simulink model "svm_stc_bldc"  (R2021a)
settings: Solver=VariableStepAuto  StartTime=0.0  StopTime=t_sim  FixedStep=t_int  MinStep=1e-6  RelTol=1e-3  EnableMultiTasking=on
InitFcn:
  | svm_stc_bldc_data
values from neighbouring files (symbols this model uses):
  b = T_nom/Q_nom    (= 6.18430636014)    [bldc_data.m]
  flux_obs_gain = 4e4    (= 40000)    [bldc_data.m]
  Id = Iq    [i_loop_data.m]
  Jm = 0.3*0.05^2    (= 0.00075)    [bldc_data.m]
  theta_obs_gain = 2e6    (= 2000000)    [bldc_data.m]
  Vcc = 360    [bldc_data.m]
undefined symbols (not defined in the file or in its folder): fluid, i_sns, Iq, p, pmsm, r, speed_obs, v_stc
libraries: mcbcontrolslib x4, simulink x2, pid_lib x1, autolibpmsmexterior x1
settings Model: Creator=Augusto  LastModifiedBy=Rodrigo
settings SolverCC: AlgebraicLoopSolver=TrustRegion  AutoInsertRateTranBlk=on
settings DataIOCC: LimitDataPoints=on  SaveFormat=Array  ReturnWorkspaceOutputs=off
settings OptimizationCC: LifeSpan=inf
settings DebuggingCC: UnderspecifiedInitializationDetection=Classic  MergeDetectMultiDrivingBlocksExec=none  SolverPrmCheckMsg=warning  SFUnexpectedBacktrackingDiag=warning  SFNoUnconditionalDefaultTransitionDiag=warning  SFExecutionAtInitializationDiag=none  ArithmeticOperatorsInVariantConditions=warning
settings HardwareCC: ProdBitPerPointer=32  ProdBitPerSizeT=32  ProdBitPerPtrDiffT=32  ProdLargestAtomicFloat=None  ProdIntDivRoundTo=Undefined  ProdEndianess=Unspecified  ProdWordSize=32  ProdHWDeviceType=32-bit Generic
settings ModelReferenceCC: PropagateSignalLabelsOutOfModel=off
settings SFSimCC: SimUseLocalCustomCode=off  CustomCodeUndefinedFunction=UseInterfaceOnly
settings RTWCC: RTWUseLocalCustomCode=off  DLArmComputeVersion=20.02.1
settings CodeAppCC: StateflowObjectComments=on
settings GRTTargetCC: TargetLangStandard=C89/C90 (ANSI)
settings ConfigComp: CovMetricSettings=dw  CovSaveCumulativeToWorkspaceVar=on  CovSaveSingleToWorkspaceVar=on  CovExternalEMLEnable=off

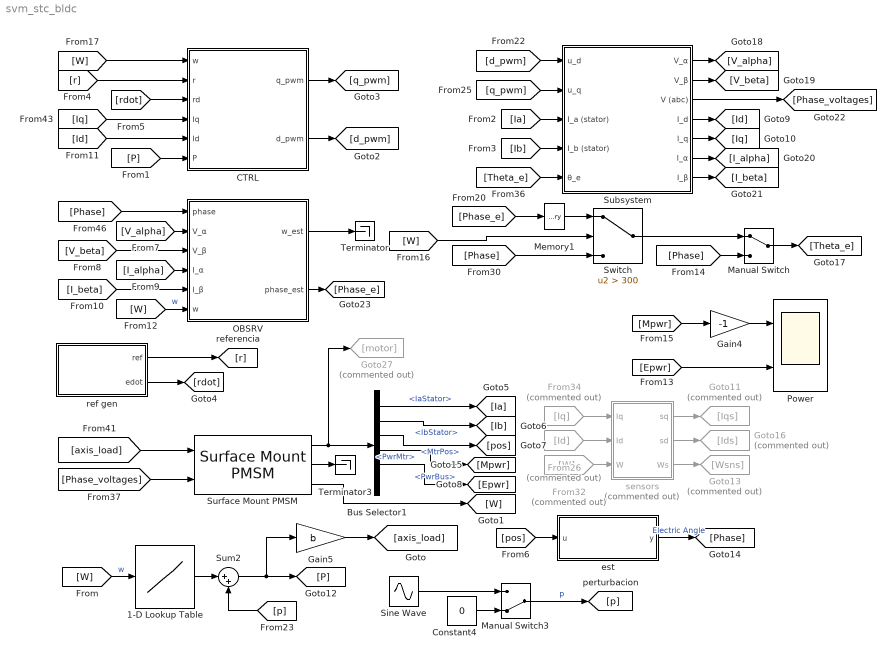
== system svm_stc_bldc ==
  1-D Lookup Table : Lookup_n-D  NumberOfTableDimensions=1  BreakpointsForDimension1=fluid.W  Table=fluid.P  InternalRulePriority=Speed  RndMeth=Simplest  InputSameDT=on
  Bus Selector1 : BusSelector  OutputSignals=IaStator,IbStator,MtrPos,PwrInfo.PwrTrnsfrd.PwrMtr,PwrInfo.PwrTrnsfrd.PwrBus,MtrSpd
  CTRL : Subsystem
  Constant4 : Constant  Value=0
  From26 : From  Commented=on  GotoTag=Id
  From32 : From  Commented=on  GotoTag=W
  From34 : From  Commented=on  GotoTag=Iq
  Gain4 : Gain  Gain=-1
  Gain5 : Gain  Gain=b
  Goto11 : Goto  Commented=on  GotoTag=Iqs
  Goto13 : Goto  Commented=on  GotoTag=Wsns
  Goto16 : Goto  Commented=on  GotoTag=Ids
  Goto27 : Goto  Commented=on  GotoTag=motor
  Manual Switch : ManualSwitch
  Manual Switch3 : ManualSwitch  CurrentSetting=0
  Memory1 : Memory
  OBSRV : Subsystem
  Power : Scope  NumInputPorts=2
  Sine Wave : Sin  Amplitude=p.a  Frequency=p.w  SampleTime=0
  Subsystem : Subsystem
  Sum2 : Sum  Inputs=|++
  Surface Mount PMSM : autolibpmsmexterior/Surface Mount PMSM  port_config=Torque  sim_type=Continuous  Ts=0.001  P=pmsm.spec.poles/2  Rs=pmsm.perf.Rs  Ldq_=pmsm.perf.L  KConstText=Permanent flux linkage constant (lambda_pm):  lambda_pm=pmsm.perf.phi  Ke=159.9771  Kt=1.323  mechanical=[Jm, 0.0001, 0.2]  idq0=[0 0]  theta_init=0  omega_init=Wo  KConst=pmsm.perf.phi  lambda_pm_calc=pmsm.perf.phi  RefBlkName='autolibpmsmexterior/Surface Mount PMSM'  aMode=5  Ldq="[0.0017      0.0017]"
      settings: SourceProductBaseCode=PW,DR,MT,UV,VE
  Switch : Switch  Criteria=u2 > Threshold  Threshold=300
  Terminator : Terminator
  Terminator3 : Terminator
  est : MATLAB Function  TreatAsAtomicUnit=on
  ref gen : Subsystem
  sensors : Subsystem  Commented=on
  wires:
  1-D Lookup Table/1 -> Sum2/1
  [p] -> Sum2/2
  Sum2/1 -> Gain5/1, [P]
  Sine Wave/1 -> Manual Switch3/1
  Manual Switch3/1 -> [p]  "p"
  Constant4/1 -> Manual Switch3/2
  [W] -> 1-D Lookup Table/1  "w"
  From34/1 -> sensors/1(Iq)
  sensors/1(sq) -> Goto11/1
  From32/1 -> sensors/3(W)
  [Phase_voltages] -> Surface Mount PMSM/2
  Bus Selector1/2 -> [Ib]  "<IbStator>"
  Subsystem/1(V_α) -> [V_alpha]
  [axis_load] -> Surface Mount PMSM/1
  [Theta_e] -> Subsystem/5(θ_e)
  Subsystem/2(V_β) -> [V_beta]
  Bus Selector1/1 -> [Ia]  "<IaStator>"
  Subsystem/6(I_α) -> [I_alpha]
  Subsystem/5(I_q) -> [Iq]
  Subsystem/7(I_β) -> [I_beta]
  Subsystem/4(I_d) -> [Id]
  est/1(y) -> [Phase]  "Electric Angle"
  Bus Selector1/3 -> [pos]  "<MtrPos>"
  Subsystem/3(V (abc)) -> [Phase_voltages]
  Surface Mount PMSM/1 -> Goto27/1, Bus Selector1/1
  Surface Mount PMSM/2 -> Terminator3/1
  Gain5/1 -> [axis_load]
  From26/1 -> sensors/2(Id)
  [Phase] -> OBSRV/1(phase)
  [d_pwm] -> Subsystem/1(u_d)
  [q_pwm] -> Subsystem/2(u_q)
  [W] -> CTRL/1(w)
  [r] -> CTRL/2(r)
  [rdot] -> CTRL/3(rd)
  [Iq] -> CTRL/4(Iq)
  [Id] -> CTRL/5(Id)
  CTRL/1(q_pwm) -> [q_pwm]
  CTRL/2(d_pwm) -> [d_pwm]
  [P] -> CTRL/6(P)
  [Ia] -> Subsystem/3(I_a (stator))
  [Ib] -> Subsystem/4(I_b (stator))
  [pos] -> est/1(u)
  sensors/2(sd) -> Goto16/1
  sensors/3(Ws) -> Goto13/1
  ref gen/1(ref) -> [r]
  ref gen/2(edot) -> [rdot]
  [V_alpha] -> OBSRV/2(V_α)
  [V_beta] -> OBSRV/3(V_β)
  [I_alpha] -> OBSRV/4(I_α)
  [I_beta] -> OBSRV/5(I_β)
  [W] -> OBSRV/6(w)  "w"
  [Epwr] -> Power/2
  [Mpwr] -> Gain4/1
  Gain4/1 -> Power/1
  Bus Selector1/5 -> [Epwr]  "<PwrBus>"
  Bus Selector1/4 -> [Mpwr]  "<PwrMtr>"
  OBSRV/2(phase_est) -> [Phase_e]
  OBSRV/1(w_est) -> Terminator/1
  [W] -> Switch/2
  Switch/1 -> Manual Switch/1
  [Phase] -> Switch/3
  Manual Switch/1 -> [Theta_e]
  [Phase] -> Manual Switch/2
  Surface Mount PMSM/3 -> [W]
  [Phase_e] -> Memory1/1
  Memory1/1 -> Switch/1

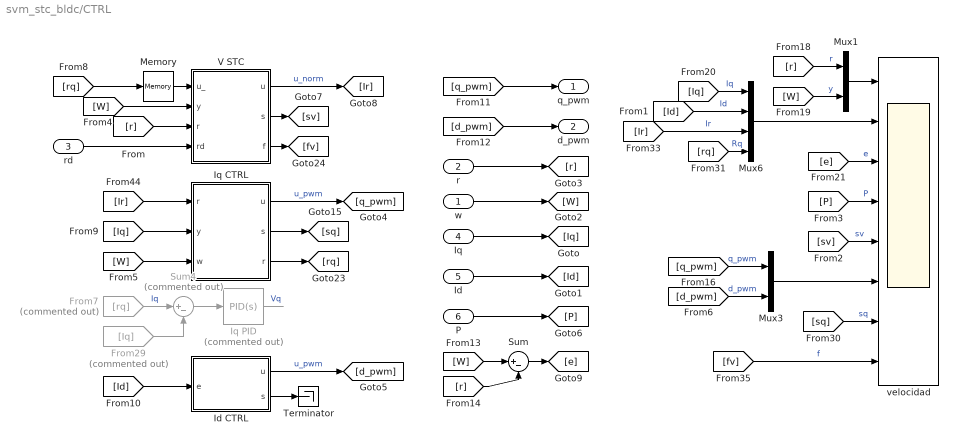
== system svm_stc_bldc/CTRL ==
  w : Inport
  r : Inport  Port=2
  rd : Inport  Port=3
  Iq : Inport  Port=4
  Id : Inport  Port=5
  P : Inport  Port=6
  From29 : From  Commented=on  GotoTag=Iq
  From7 : From  Commented=on  GotoTag=rq
  Id CTRL : MATLAB Function  TreatAsAtomicUnit=on  SystemSampleTime=Id.ts
  Iq CTRL : MATLAB Function  TreatAsAtomicUnit=on  SystemSampleTime=Iq.ts
  Iq PID : pid_lib/PID Controller  Commented=on  Controller=PID  Form=Parallel  TimeDomain=Continuous-time  UseExternalTs=off  SampleTime=-1  IntegratorMethod=Forward Euler  FilterMethod=Forward Euler  ControllerParametersSource=internal  P=10/Vcc  I=100/Vcc  D=1/Vcc  UseFilter=on  N=100  TunerSelectOption=Transfer Function Based (PID Tuner App)  InitialConditionSource=internal  InitialConditionForIntegrator=0  InitialConditionForFilter=0  DifferentiatorICPrevScaledInput=0  ExternalReset=none  TrackingMode=off  Kt=1  LimitOutput=on  SatLimitsSource=internal  UpperSaturationLimit=Vcc  LowerSaturationLimit=-Vcc  LinearizeAsGain=on  AntiWindupMode=back-calculation  Kb=1  POutMin=[]  POutMax=[]  IOutMin=[]  IOutMax=[]  DOutMin=[]  DOutMax=[]  NOutMin=[]  NOutMax=[]  SumOutMin=[]  SumOutMax=[]  SaturationOutMin=[]  SaturationOutMax=[]  PParamMin=[]  PParamMax=[]  IParamMin=[]  IParamMax=[]  DParamMin=[]  DParamMax=[]  NParamMin=[]  NParamMax=[]  KbParamMin=[]  KbParamMax=[]  KtParamMin=[]  KtParamMax=[]  KbOutMin=[]  KbOutMax=[]  KtOutMin=[]  KtOutMax=[]  IntegratorOutMin=[]  IntegratorOutMax=[]  FilterOutMin=[]  FilterOutMax=[]  SumI1OutMin=[]  SumI1OutMax=[]  SumI2OutMin=[]  SumI2OutMax=[]  SumI3OutMin=[]  SumI3OutMax=[]  SumI4OutMin=[]  SumI4OutMax=[]  SumDOutMin=[]  SumDOutMax=[]  DifferentiatorOutMin=[]  DifferentiatorOutMax=[]  FilterDiffOutCoefMin=[]  FilterDiffOutCoefMax=[]  ReciprocalOutMin=[]  ReciprocalOutMax=[]  SumDenOutMin=[]  SumDenOutMax=[]  SumNumOutMin=[]  SumNumOutMax=[]  DivideOutMin=[]  DivideOutMax=[]  UdiffTsProdOutMin=[]  UdiffTsProdOutMax=[]  NTsProdOutMin=[]  NTsProdOutMax=[]  UintegralTsProdOutMin=[]  UintegralTsProdOutMax=[]  UngainTsProdOutMin=[]  UngainTsProdOutMax=[]  IntegratorContinuousStateAttributes=''  IntegratorStateMustResolveToSignalObject=off  IntegratorRTWStateStorageClass=Auto  FilterContinuousStateAttributes=''  FilterStateMustResolveToSignalObject=off  FilterRTWStateStorageClass=Auto  ParallelPVariant=InternalParameters  IdealPVariant=Disabled  IVariant=InternalParameters  DVariant=InternalParameters  IntegratorVariant=Continuous  SatVariant=Enabled  AWVariant=BackCalculation  PCopyVariant=Disabled  TRVariant=Disabled  FdbkBlocksVariant=Forward  IdealPFdbkVariant=Disabled  SatFdbkVariant=Disabled  DerivativeFilterVariant=ContFilter  NVariant=InternalParameters  NCopyVariant=Disabled  FilterICVariant=InternalICsFilter  IntegratorICVariant=InternalICs  ExternalResetVariant=Disabled  TRSumVariant=Passthrough  SumFdbkVariant=Disabled  SumVariant=Sum_PID  TsampFilterVariant=InternalTs  TsampNgainVariant=Passthrough  TsampIntegralVariant=Passthrough  ExternalSaturationOutDataTypeStr=Inherit: Same as second input
  Memory : Memory
  Mux1 : Mux  Inputs=2
  Mux3 : Mux  Inputs=2
  Mux6 : Mux
  Sum : Sum  Inputs=|+-
  Sum4 : Sum  Commented=on  Inputs=|+-
  Terminator : Terminator
  V STC : MATLAB Function  TreatAsAtomicUnit=on  SystemSampleTime=v_stc.ts
  velocidad : Scope  NumInputPorts=8
  q_pwm : Outport
  d_pwm : Outport  Port=2
  wires:
  V STC/3(f) -> [fv]
  Sum4/1 -> Iq PID/1
  From29/1 -> Sum4/2
  Id/1 -> [Id]
  V STC/2(s) -> [sv]
  Memory/1 -> V STC/1(u_)
  Id CTRL/1(u) -> [d_pwm]  "u_pwm"
  [Ir] -> Iq CTRL/1("r ")
  r/1 -> [r]
  Iq CTRL/1(u) -> [q_pwm]  "u_pwm"
  [rq] -> Memory/1
  Iq PID/1 -> ?  "Vq"
  Iq CTRL/3(r) -> [rq]
  w/1 -> [W]
  From7/1 -> Sum4/1  "Iq"
  V STC/1(u) -> [Ir]  "u_norm"
  Id CTRL/2(s) -> Terminator/1
  Iq/1 -> [Iq]
  rd/1 -> V STC/4(rd)
  Iq CTRL/2(s) -> [sq]
  [sq] -> velocidad/7  "sq"
  [sv] -> velocidad/5  "sv"
  [W] -> Mux1/2  "y"
  [rq] -> Mux6/4  "Rq"
  [P] -> velocidad/4  "P"
  [d_pwm] -> Mux3/2  "d_pwm"
  [e] -> velocidad/3  "e"
  [Ir] -> Mux6/3  "Ir"
  [Id] -> Mux6/2  "Id"
  Mux6/1 -> velocidad/2
  [fv] -> velocidad/8  "f"
  Mux1/1 -> velocidad/1
  [q_pwm] -> Mux3/1  "q_pwm"
  [r] -> Mux1/1  "r"
  Mux3/1 -> velocidad/6
  [Iq] -> Mux6/1  "Iq"
  [r] -> V STC/3(r)
  [W] -> V STC/2(y)
  [W] -> Iq CTRL/3(w)
  [Iq] -> Iq CTRL/2(y)
  [Id] -> Id CTRL/1(e)
  [q_pwm] -> q_pwm/1
  [d_pwm] -> d_pwm/1
  P/1 -> [P]
  Sum/1 -> [e]
  [W] -> Sum/1
  [r] -> Sum/2

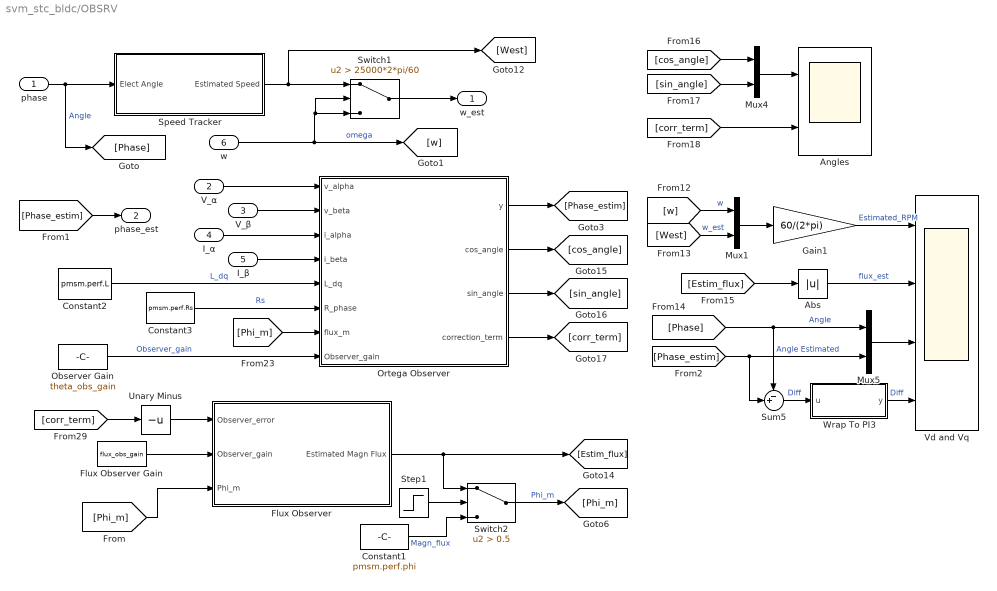
== system svm_stc_bldc/OBSRV ==
  phase : Inport
  V_α : Inport  Port=2
  V_β : Inport  Port=3
  I_α : Inport  Port=4
  I_β : Inport  Port=5
  w : Inport  Port=6
  Abs : Abs
  Angles : Scope  NumInputPorts=2
  Constant1 : Constant  Value=pmsm.perf.phi
  Constant2 : Constant  Value=pmsm.perf.L
  Constant3 : Constant  Value=pmsm.perf.Rs
  Flux Observer : Subsystem
  Flux Observer Gain : Constant  Value=flux_obs_gain
  Gain1 : Gain  Gain=60/(2*pi)
  Mux1 : Mux  Inputs=2
  Mux4 : Mux  Inputs=2
  Mux5 : Mux  Inputs=2
  Observer Gain : Constant  Value=theta_obs_gain
  Ortega Observer : Subsystem
  Speed Tracker : Subsystem
  Step1 : Step  Time=0.01  After=2  SampleTime=0
  Sum5 : Sum  Inputs=-+|
  Switch1 : Switch  Criteria=u2 > Threshold  Threshold=25000*2*pi/60
  Switch2 : Switch  Criteria=u2 > Threshold  Threshold=0.5
  Unary Minus : UnaryMinus
  Vd and Vq : Scope  NumInputPorts=4
  Wrap To PI3 : MATLAB Function  TreatAsAtomicUnit=on
  w_est : Outport
  phase_est : Outport  Port=2
  wires:
  Switch1/1 -> w_est/1
  [Phi_m] -> Ortega Observer/7(flux_m)
  V_β/1 -> Ortega Observer/2(v_beta)
  Ortega Observer/3(sin_angle) -> [sin_angle]
  Constant2/1 -> Ortega Observer/5(L_dq)  "L_dq"
  Constant3/1 -> Ortega Observer/6(R_phase)  "Rs"
  Ortega Observer/1(y) -> [Phase_estim]
  Ortega Observer/2(cos_angle) -> [cos_angle]
  Flux Observer/1(Estimated Magn Flux) -> Switch2/1, [Estim_flux]
  Constant1/1 -> Switch2/3  "Magn_flux"
  Unary Minus/1 -> Flux Observer/1(Observer_error)
  Step1/1 -> Switch2/2
  Flux Observer Gain/1 -> Flux Observer/2(Observer_gain)
  Observer Gain/1 -> Ortega Observer/8(Observer_gain)  "Observer_gain"
  V_α/1 -> Ortega Observer/1(v_alpha)
  Ortega Observer/4(correction_term) -> [corr_term]
  Switch2/1 -> [Phi_m]  "Phi_m"
  [corr_term] -> Unary Minus/1
  I_α/1 -> Ortega Observer/3(i_alpha)
  I_β/1 -> Ortega Observer/4(i_beta)
  phase/1 -> [Phase], Speed Tracker/1(Elect Angle)  "Angle"
  [Phi_m] -> Flux Observer/3(Phi_m)
  Mux4/1 -> Angles/1
  [w] -> Mux1/1  "w"
  [sin_angle] -> Mux4/2
  [cos_angle] -> Mux4/1
  [West] -> Mux1/2  "w_est"
  Abs/1 -> Vd and Vq/2  "flux_est"
  [Estim_flux] -> Abs/1
  [corr_term] -> Angles/2
  Mux1/1 -> Gain1/1
  [Phase_estim] -> phase_est/1
  Speed Tracker/1(Estimated Speed) -> [West], Switch1/1
  Gain1/1 -> Vd and Vq/1  "Estimated_RPM"
  [Phase] -> Sum5/1, Mux5/1  "Angle"
  Mux5/1 -> Vd and Vq/3
  [Phase_estim] -> Sum5/2, Mux5/2  "Angle Estimated"
  Sum5/1 -> Wrap To PI3/1(u)  "Diff"
  Wrap To PI3/1(y) -> Vd and Vq/4  "Diff"
  w/1 -> [w], Switch1/3, Switch1/2  "omega"

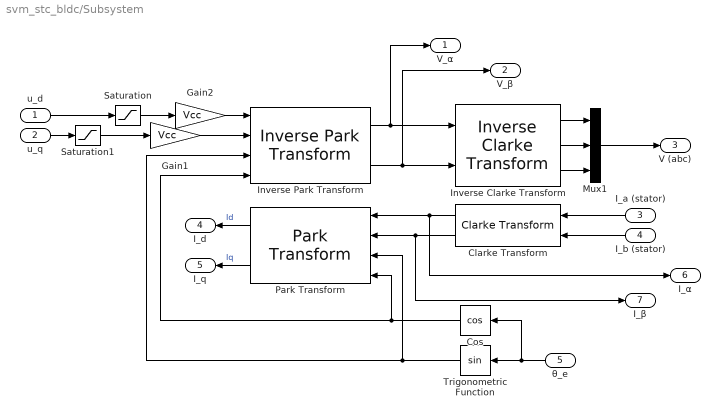
== system svm_stc_bldc/Subsystem ==
  u_d : Inport
  u_q : Inport  Port=2
  I_a (stator) : Inport  Port=3
  I_b (stator) : Inport  Port=4
  θ_e : Inport  Port=5
  Clarke Transform : mcbcontrolslib/Clarke Transform  VariantControl=Variant2
  Cos : Trigonometry  Operator=cos
  Gain1 : Gain  Gain=Vcc
  Gain2 : Gain  Gain=Vcc
  Inverse Clarke Transform : mcbcontrolslib/Inverse Clarke Transform
      settings: SourceProductBaseCode=MT
  Inverse Park Transform : mcbcontrolslib/Inverse Park Transform  AxisAlignment=D-axis
  Mux1 : Mux  Inputs=3
  Park Transform : mcbcontrolslib/Park Transform  AxisAlignment=D-axis
      settings: SourceProductBaseCode=MT
  Saturation : Saturate  UpperLimit=0.95  LowerLimit=-0.95
  Saturation1 : Saturate  UpperLimit=0.95  LowerLimit=-0.95
  Trigonometric Function : Trigonometry
  V_α : Outport
  V_β : Outport  Port=2
  V (abc) : Outport  Port=3
  I_d : Outport  Port=4
  I_q : Outport  Port=5
  I_α : Outport  Port=6
  I_β : Outport  Port=7
  wires:
  I_b (stator)/1 -> Clarke Transform/2
  Mux1/1 -> V (abc)/1
  u_q/1 -> Saturation1/1
  I_a (stator)/1 -> Clarke Transform/1
  Clarke Transform/2 -> I_β/1, Park Transform/2
  Cos/1 -> Park Transform/4, Inverse Park Transform/4
  Clarke Transform/1 -> I_α/1, Park Transform/1
  θ_e/1 -> Cos/1, Trigonometric Function/1
  Park Transform/2 -> I_q/1  "Iq"
  Inverse Park Transform/2 -> V_β/1, Inverse Clarke Transform/2
  Park Transform/1 -> I_d/1  "Id"
  Inverse Clarke Transform/2 -> Mux1/2
  Trigonometric Function/1 -> Park Transform/3, Inverse Park Transform/3
  u_d/1 -> Saturation/1
  Inverse Park Transform/1 -> V_α/1, Inverse Clarke Transform/1
  Inverse Clarke Transform/3 -> Mux1/3
  Inverse Clarke Transform/1 -> Mux1/1
  Gain2/1 -> Inverse Park Transform/1
  Gain1/1 -> Inverse Park Transform/2
  Saturation/1 -> Gain2/1
  Saturation1/1 -> Gain1/1

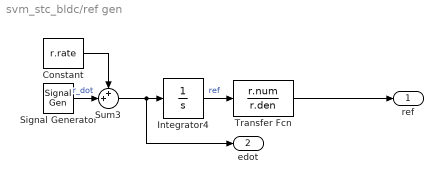
== system svm_stc_bldc/ref gen ==
  Constant : Constant  Value=r.rate
  Integrator4 : Integrator  InitialCondition=r.off  LimitOutput=on  UpperSaturationLimit=r.lim  LowerSaturationLimit=0
  Signal Generator : SignalGenerator  Amplitude=r.a  Frequency=r.f
  Sum3 : Sum  Inputs=++|
  Transfer Fcn : TransferFcn  Numerator=r.num  Denominator=r.den
  ref : Outport
  edot : Outport  Port=2
  wires:
  Constant/1 -> Sum3/1
  Signal Generator/1 -> Sum3/2  "r_dot"
  Sum3/1 -> edot/1, Integrator4/1
  Transfer Fcn/1 -> ref/1
  Integrator4/1 -> Transfer Fcn/1  "ref"

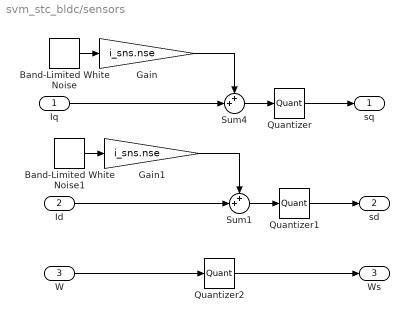
== system svm_stc_bldc/sensors ==
  Iq : Inport
  Id : Inport  Port=2
  W : Inport  Port=3
  Band-Limited White Noise : simulink/Sources/Band-Limited White Noise  Cov=Iq.ts  Ts=Iq.ts  seed=[29841]
  Band-Limited White Noise1 : simulink/Sources/Band-Limited White Noise  Cov=Iq.ts  Ts=Iq.ts  seed=[29841]
  Gain : Gain  Gain=i_sns.nse
  Gain1 : Gain  Gain=i_sns.nse
  Quantizer : Quantizer  QuantizationInterval=i_sns.qnt
  Quantizer1 : Quantizer  QuantizationInterval=i_sns.qnt
  Quantizer2 : Quantizer  QuantizationInterval=w_sns.qnt
  Sum1 : Sum  Inputs=++|
  Sum4 : Sum  Inputs=++|
  sq : Outport
  sd : Outport  Port=2
  Ws : Outport  Port=3
  wires:
  Iq/1 -> Sum4/2
  Band-Limited White Noise/1 -> Gain/1
  Sum4/1 -> Quantizer/1
  Quantizer/1 -> sq/1
  Gain/1 -> Sum4/1
  Band-Limited White Noise1/1 -> Gain1/1
  Quantizer1/1 -> sd/1
  Id/1 -> Sum1/2
  Sum1/1 -> Quantizer1/1
  Gain1/1 -> Sum1/1
  W/1 -> Quantizer2/1
  Quantizer2/1 -> Ws/1

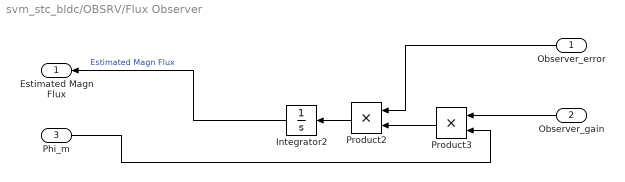
== system svm_stc_bldc/OBSRV/Flux Observer ==
  Observer_error : Inport
  Observer_gain : Inport  Port=2
  Phi_m : Inport  Port=3
  Integrator2 : Integrator
  Product2 : Product
  Product3 : Product
  Estimated Magn Flux : Outport
  wires:
  Product3/1 -> Product2/2
  Product2/1 -> Integrator2/1
  Observer_error/1 -> Product2/1
  Observer_gain/1 -> Product3/1
  Phi_m/1 -> Product3/2
  Integrator2/1 -> Estimated Magn Flux/1  "Estimated Magn Flux"

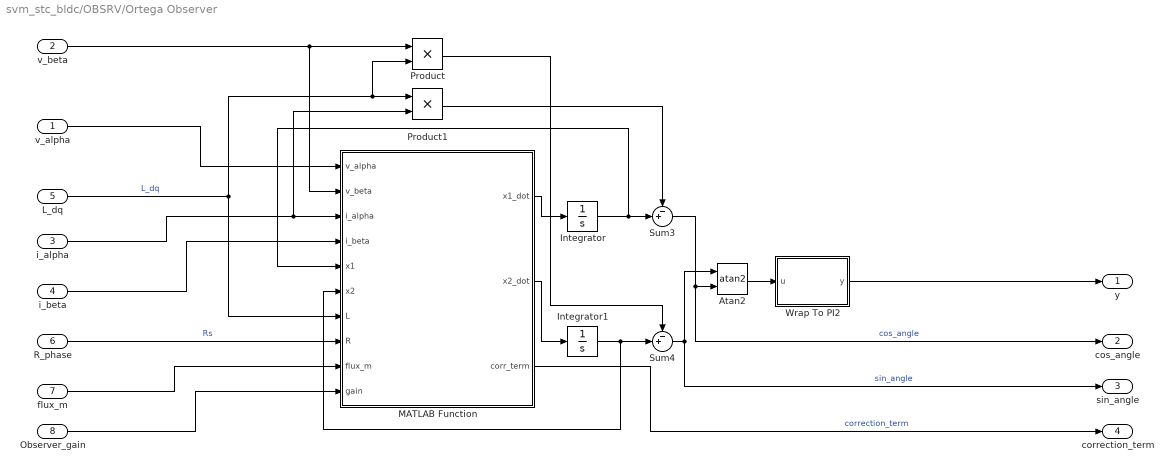
== system svm_stc_bldc/OBSRV/Ortega Observer ==
  v_alpha : Inport
  v_beta : Inport  Port=2
  i_alpha : Inport  Port=3
  i_beta : Inport  Port=4
  L_dq : Inport  Port=5
  R_phase : Inport  Port=6
  flux_m : Inport  Port=7
  Observer_gain : Inport  Port=8
  Atan2 : Trigonometry  Operator=atan2
  Integrator : Integrator
  Integrator1 : Integrator
  MATLAB Function : MATLAB Function  TreatAsAtomicUnit=on
  Product : Product
  Product1 : Product
  Sum3 : Sum  Inputs=-+|
  Sum4 : Sum  Inputs=-+|
  Wrap To PI2 : MATLAB Function  TreatAsAtomicUnit=on
  y : Outport
  cos_angle : Outport  Port=2
  sin_angle : Outport  Port=3
  correction_term : Outport  Port=4
  wires:
  i_alpha/1 -> MATLAB Function/3(i_alpha), Product1/2
  L_dq/1 -> MATLAB Function/7(L), Product/2, Product1/1  "L_dq"
  Integrator1/1 -> Sum4/2, MATLAB Function/6(x2)
  MATLAB Function/1(x1_dot) -> Integrator/1
  v_beta/1 -> MATLAB Function/2(v_beta), Product/1
  Atan2/1 -> Wrap To PI2/1(u)
  Product/1 -> Sum4/1
  Wrap To PI2/1(y) -> y/1
  Integrator/1 -> Sum3/2, MATLAB Function/5(x1)
  Sum4/1 -> sin_angle/1, Atan2/1  "sin_angle"
  Sum3/1 -> cos_angle/1, Atan2/2  "cos_angle"
  Product1/1 -> Sum3/1
  MATLAB Function/3(corr_term) -> correction_term/1  "correction_term"
  flux_m/1 -> MATLAB Function/9(flux_m)
  Observer_gain/1 -> MATLAB Function/10(gain)
  R_phase/1 -> MATLAB Function/8(R)  "Rs"
  MATLAB Function/2(x2_dot) -> Integrator1/1
  i_beta/1 -> MATLAB Function/4(i_beta)
  v_alpha/1 -> MATLAB Function/1(v_alpha)

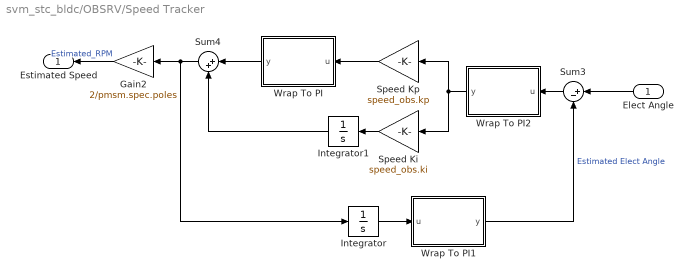
== system svm_stc_bldc/OBSRV/Speed Tracker ==
  Elect Angle : Inport
  Gain2 : Gain  Gain=2/pmsm.spec.poles
  Integrator : Integrator
  Integrator1 : Integrator
  Speed Ki : Gain  Gain=speed_obs.ki
  Speed Kp : Gain  Gain=speed_obs.kp
  Sum3 : Sum  Inputs=|+-
  Sum4 : Sum  Inputs=|++
  Wrap To PI : MATLAB Function  TreatAsAtomicUnit=on
  Wrap To PI1 : MATLAB Function  TreatAsAtomicUnit=on
  Wrap To PI2 : MATLAB Function  TreatAsAtomicUnit=on
  Estimated Speed : Outport
  wires:
  Speed Ki/1 -> Integrator1/1
  Integrator1/1 -> Sum4/2
  Sum4/1 -> Gain2/1, Integrator/1
  Integrator/1 -> Wrap To PI1/1(u)
  Wrap To PI/1(y) -> Sum4/1
  Speed Kp/1 -> Wrap To PI/1(u)
  Wrap To PI1/1(y) -> Sum3/2  "Estimated Elect Angle"
  Elect Angle/1 -> Sum3/1
  Sum3/1 -> Wrap To PI2/1(u)
  Wrap To PI2/1(y) -> Speed Kp/1, Speed Ki/1
  Gain2/1 -> Estimated Speed/1  "Estimated_RPM"

== matlab function svm_stc_bldc/OBSRV/Ortega Observer/Wrap To PI2 ==
  data: u input; y output
function y = fcn(u)

y = wrapToPi(u);

== matlab function svm_stc_bldc/OBSRV/Speed Tracker/Wrap To PI ==
  data: u input; y output
function y = fcn(u)

y = wrapToPi(u);

== matlab function svm_stc_bldc/OBSRV/Speed Tracker/Wrap To PI1 ==
  data: u input; y output
function y = fcn(u)

y = wrapToPi(u);

== matlab function svm_stc_bldc/OBSRV/Speed Tracker/Wrap To PI2 ==
  data: u input; y output
function y = fcn(u)

y = wrapToPi(u);

== matlab function svm_stc_bldc/OBSRV/Wrap To PI3 ==
  data: u input; y output
function y = fcn(u)

y = wrapToPi(u);

== matlab function svm_stc_bldc/CTRL/V STC ==
  data: u_ input; y input size=1; r input size=1; rd input; u output size=1; s output size=1; v_stc parameter size=1; f output
% r : referencia
% y : medicion
% u_: accion de control precedente
% stc: configuracion (cargada en el workspace) con campos 
%      .l1 : ganancia proporcional
%      .l2 : ganancia integral
%      .ts : tiempo de muestreo

function [u, s, f] = vel_dstc(u_, y, r, rd, v_stc) 
    persistent up ff e_ % componente proporcional
    e  = (y - r)/v_stc.e_norm;   % variable de deslizamiento
    if isempty(up)
        up = 0;
        ff = 0;
        e_ = e;
    end
    ui = (u_/v_stc.u_norm - ff)/v_stc.bu - up;
    if sign(ui) ~= sign(u_)
        ui = 0;
    end

    if v_stc.k2 > 0
        e_dot = (e - e_)/v_stc.ts;
        e_ = e;
        s = v_stc.k2*sabs(e,2/3) + e_dot;
    else
        s = e;
    end
    ff = v_stc.bf*rd;
    [l1, l2, f] = st_gains(s, v_stc);    
    [up, ui] = dstc_imp(ui, s, l1, l2, v_stc.ts);
    u = (up + ui)*v_stc.bu + ff;
    % u = us;  % accion de control
    % r = u - u_;
    % if abs(r) > v_stc.Ur
    %     u = u_ + sign(r) * v_stc.Ur;
    % end
    if abs(u) > v_stc.UM
        u = v_stc.UM * sign(u);
    end
    % if u ~= us
    %     ui = (u-ff)/v_stc.bu - up;
    %     if sign(ui) ~= sign(u)
    %         ui = 0;
    %     end
    % end
    u = u * v_stc.u_norm;
end 

% up: parte proporcional
% ui: parte integral
function [up, ui] = dstc_imp(ui, s, l1, l2, ts) 
    a    = ts* l1;
    hl2  = ts* l2;
    h2l2 = hl2 * ts;
    bk = -s - ts*ui;
    if     bk <-h2l2
        z  = (sqrt(a^2 - 4*(bk + h2l2))-a)/2;
        ui =  ui - hl2;
        up = -l1*z;
    elseif bk > h2l2
        z  = (sqrt(a^2 + 4*(bk - h2l2))-a)/2;
        ui =  ui + hl2;
        up =  l1*z;
    else
        ui = -s / ts;
        up =  0;
    end
end
% function [up, ui] = dstc_exp(ui, s, l1, l2, ts) 
%     up = -l1*sabs(s,0.5);
%     ui =  ui - l2*sign(s)*ts;
% end
function [l1, l2, f] = st_gains(s, cfg)
    e  = abs(s);
    if  e < cfg.e_tol
        f = sqrt(e/cfg.e_tol);
    elseif cfg.e_b > 0 && e > cfg.e_bar
        e = e - cfg.e_bar;
        if  e < cfg.e_mu
            e = cfg.e_mu - e;
            f = cfg.e_b * sqrt(cfg.e_mu/e);
            if  f > cfg.f_max
                f = cfg.f_max;
            end
        else
            f = cfg.f_max;
        end
    else
        f = 1;
    end
    l1 = cfg.l1 * f;
    l2 = cfg.l2 * f*f;
end

function s = sabs(x, p)
    if x == 0
        s = 0;
    else
        s = sign(x) * abs(x)^p;    
    end
end

== matlab function svm_stc_bldc/CTRL/Id CTRL ==
  data: e input size=1; u output size=1; s output size=1; Id parameter
% r : referencia
% y : medicion
% u_: accion de control precedente
% stc: configuracion (cargada en el workspace) con campos 
%      .l1 : ganancia proporcional
%      .l2 : ganancia integral
%      .ts : tiempo de muestreo

function [u, s] = id_loop(e, Id) 
    persistent ui e_ e_dot % componente proporcional
    if isempty(e_)
        ui = 0;
        e_ = e;
        e_dot = 0;
    end
    e_dot = (e - e_)*Id.f1 + e_dot*Id.f2;
    e_ = e;

    if Id.pid.kp > 0
        [u_, up] = PID(-e, -e_dot, ui, Id.pid);
        s = 0;
    else
        [u_, up, s] = STC(e, ui, Id.stc, Id.ts);
    end
    u  = u_*Id.bu;  % accion de control
    % saturacion y anti-windup
    if abs(u) > Id.UM
        u  = sign(u) * Id.UM;
        u_ = u/Id.bu;  % accion de control
    end
    ui = u_ - up;
    % if sign(ui) ~= sign(u_) 
    %     ui = 0;
    % end
end 

%%
function [u, up] = PID(e, e_dot, ui, cfg) 
    up = cfg.kp * e + cfg.kd * e_dot;
    u  = up + ui + cfg.ki_ts * e;
end 
function [u, up, s] = STC(e, ui, cfg, ts) 
    s  = -e;   % variable de deslizamiento
    [l1, l2] = st_gains(s, cfg);  
    [up, ui] = dstc_imp(ui, s, l1, l2, ts);
    u = up + ui;
end 

% up: parte proporcional
% ui: parte integral
function [up, ui] = dstc_imp(ui, s, l1, l2, ts) 
    a    = ts* l1;
    hl2  = ts* l2;
    h2l2 = hl2 * ts;
    bk = -s - ts*ui;
    if     bk <-h2l2
        z  = (sqrt(a^2 - 4*(bk + h2l2))-a)/2;
        ui =  ui - hl2;
        up = -l1*z;
    elseif bk > h2l2
        z  = (sqrt(a^2 + 4*(bk - h2l2))-a)/2;
        ui =  ui + hl2;
        up =  l1*z;
    else
        ui = -s/ts;
        up = 0;
    end
end
% function [up, ui] = dstc_exp(ui, s, l1, l2, ts) 
%     up = -l1*sabs(s,0.5);
%     ui =  ui - l2*sign(s)*ts;
% end
function [l1, l2, f] = st_gains(s, cfg)
    e  = abs(s);
    if  e < cfg.e_tol
        f = sqrt(e/cfg.e_tol);
    elseif cfg.e_b > 0 && e > cfg.e_bar
        e = e - cfg.e_bar;
        if  e < cfg.e_mu
            e = cfg.e_mu - e;
            f = cfg.e_b * sqrt(cfg.e_mu/e);
            if  f > cfg.f_max
                f = cfg.f_max;
            end
        else
            f = cfg.f_max;
        end
    else
        f = 1;
    end
    l1 = cfg.l1 * f;
    l2 = cfg.l2 * f*f;
end

function s = sabs(x, p)
    if x == 0
        s = 0;
    else
        s = sign(x) * abs(x)^p;    
    end
end

== matlab function svm_stc_bldc/CTRL/Iq CTRL ==
  data: r input size=1; y input size=1; w input; u output size=1; s output size=1; Iq parameter; r output
% r : referencia
% y : medicion
% u_: accion de control precedente
% stc: configuracion (cargada en el workspace) con campos 
%      .l1 : ganancia proporcional
%      .l2 : ganancia integral
%      .ts : tiempo de muestreo

function [u, s, r] = iq_loop(r, y, w, Iq) 
    persistent up e_ r_ u_ % componente proporcional
    if isempty(e_)
        up = 0;
        e_ = 0;
        r_ = 0;
        u_ = 0;
    end
    dr = r - r_;
    if abs(dr) > Iq.rlim
        r = r_ + sign(dr)*Iq.rlim;
    end
    r_ = r;
    e  = r - y;   % variable de deslizamiento
    e_dot = (e - e_)/Iq.ts;
    e_ = e;

    ui = u_ - up;
    if sign(ui) ~= sign(u_) 
        ui = 0;
    end
    
    if Iq.pid.kp > 0
        [u_, up] = PID(e, e_dot, ui, Iq.pid);
        s = 0;
    else
        [u_, up, s] = STC(e, e_dot, ui, Iq.stc, Iq.ts);
    end
    ff = Iq.bd * y + Iq.bf * w;
    
    u  = u_*Iq.bu + ff;  % accion de control
    % saturacion y anti-windup
    if abs(u) > Iq.UM
        u  = sign(u) * Iq.UM;
        u_ = (u - ff)/Iq.bu;  % accion de control
    end
end 

function [u, up] = PID(e, e_dot, ui, cfg) 
    up = cfg.kp * e + cfg.kd * e_dot;
    u  = up + ui + cfg.ki_ts * e;
end 
function [u, up, s] = STC(e, e_dot, ui, cfg, ts)     
    if cfg.k2 > 0
        s  = cfg.k2*sabs(e,2/3) + e_dot;
    else
        s = e;
    end    
    [l1, l2] = st_gains(s, cfg);  
    [up, ui] = dstc_imp(ui, s, l1, l2, ts);
    u = up + ui;
end 

% up: parte proporcional
% ui: parte integral
function [up, ui] = dstc_imp(ui, s, l1, l2, ts) 
    a    = ts* l1;
    hl2  = ts* l2;
    h2l2 = hl2 * ts;
    bk = -s - ts*ui;
    if     bk <-h2l2
        z  = (sqrt(a^2 - 4*(bk + h2l2))-a)/2;
        ui =  ui - hl2;
        up = -l1*z;
    elseif bk > h2l2
        z  = (sqrt(a^2 + 4*(bk - h2l2))-a)/2;
        ui =  ui + hl2;
        up =  l1*z;
    else
        ui = -s/ts;
        up = 0;
    end
end
function [up, ui] = dstc_exp(ui, s, l1, l2, ts) 
    up = -l1*sabs(s,0.5);
    ui =  ui - l2*sign(s)*ts;
end
function [l1, l2, f] = st_gains(s, cfg)
    e  = abs(s);
    if  e < cfg.e_tol
        f = sqrt(e/cfg.e_tol);
    elseif cfg.e_b > 0 && e > cfg.e_bar
        e = e - cfg.e_bar;
        if  e < cfg.e_mu
            e = cfg.e_mu - e;
            f = cfg.e_b * sqrt(cfg.e_mu/e);
            if  f > cfg.f_max
                f = cfg.f_max;
            end
        else
            f = cfg.f_max;
        end
    else
        f = 1;
    end
    l1 = cfg.l1 * f;
    l2 = cfg.l2 * f*f;
end

function s = sabs(x, p)
    if x == 0
        s = 0;
    else
        s = sign(x) * abs(x)^p;    
    end
end

== matlab function svm_stc_bldc/est ==
  data: u input; y output; pmsm parameter
function y = phase_from_pos(u,pmsm)

y = wrapToPi(u*pmsm.spec.poles/2);

== matlab function svm_stc_bldc/OBSRV/Ortega Observer/MATLAB Function ==
  data: v_alpha input; x1_dot output; v_beta input; i_alpha input; i_beta input; x2_dot output; x1 input; x2 input; L input; R input; flux_m input; gain input; corr_term output
function [x1_dot,x2_dot,corr_term] = ortega_obs(v_alpha, v_beta, i_alpha, i_beta, x1, x2, L, R, flux_m, gain)

corr_term = flux_m^2 - ((x1 - L*i_alpha)^2 + (x2 - L*i_beta)^2);

% if(corr_term < 0)
%      corr_term = 0;
% end

x1_dot = v_alpha - R*i_alpha + gain/2 * (x1 - L*i_alpha) * corr_term;
x2_dot = v_beta - R*i_beta + gain/2 * (x2 - L*i_beta) * corr_term;
